simulink model "uz_codegen_mtpa_me"  (R2022b)
settings: Solver=FixedStepDiscrete  StartTime=0.0  StopTime=50  RelTol=1e-3  EnableMultiTasking=on
PreLoadFcn:
  | uz_setCodegenPaths
model workspace (MATLAB code in the model file):
  | cmdLim = Simulink.Parameter;
  | cmdLim.Value = 15;
  | cmdLim.Description = 'Limit for controlling the maximum surface command angle.';
  | cmdLim.Min = 0;
  | cmdLim.Max = 90;
  | cmdLim.DocUnits = 'deg';
  | 
  | dispGain = Simulink.Parameter;
  | dispGain.Value = 0.75;
  | dispGain.Description = 'Gain applied to the displacement error.';
  | dispGain.Min = 0;
  | dispGain.Max = [];
  | dispGain.DocUnits = 'deg/sec/deg';
  | 
  | dispLim = Simulink.Parameter;
  | dispLim.Value = 30;
  | dispLim.Description = 'Limit for controlling the maximum commanded angle.';
  | dispLim.Min = 0;
  | dispLim.Max = 180;
  | dispLim.DocUnits = 'deg';
  | 
  | intGain = Simulink.Parameter;
  | intGain.Value = 0.5;
  | intGain.Description = 'Gain applied to the integral error.';
  | intGain.Min = 0;
  | intGain.Max = [];
  | intGain.DocUnits = 'deg/sec/deg/sec';
  | 
  | intLim = Simulink.Parameter;
  | intLim.Value = 5;
  | intLim.Description = 'Limit for controlling the maximum commanded angle.';
  | intLim.Min = 0;
  | intLim.Max = 90;
  | intLim.DocUnits = 'deg';
  | 
  | rateGain = Simulink.Parameter;
  | rateGain.Value = 2;
  | rateGain.Description = 'Gain applied to the rate error.';
  | rateGain.Min = 0;
  | rateGain.Max = [];
  | rateGain.DocUnits = 'deg/deg/sec';
  | 
  | rateLim = Simulink.Parameter;
  | rateLim.Value = 6;
  | rateLim.Description = 'Limit for controlling the maximum commanded angle.';
  | rateLim.Min = 0;
  | rateLim.Max = 180;
  | rateLim.DocUnits = 'deg/sec';
  | 
  | hdgGain = Simulink.Parameter;
  | hdgGain.Value = 0.015;
undefined symbols (not defined in the file or in its folder): id_ME, id_MTPA, iq_ME, iq_MTPA, M_Mi_ME, M_Mi_MTPA, omega_ME
settings Model: RequirementInfo={} %GIDa_fe9045fd_0412_4b6e_8206_617cc20e6fde  FPTRunName=Active  Creator=ts  LastModifiedBy=Nina Diringer
settings SolverCC: AlgebraicLoopSolver=TrustRegion  PositivePriorityOrder=on  AutoInsertRateTranBlk=on
settings DataIOCC: SaveOutput=off  SignalLogging=off  DSMLogging=off  SaveTime=off
settings OptimizationCC: DefaultParameterBehavior=Inlined  UseDivisionForNetSlopeComputation=on  GainParamInheritBuiltInType=on  UseFloatMulNetSlope=on  UseSpecifiedMinMax=on  InlineInvariantSignals=on  PassReuseOutputArgsAs=Individual arguments  NoFixptDivByZeroProtection=on  EfficientFloat2IntCast=on  LifeSpan=1  MaxStackSize=64  OptimizeBlockOrder=speed  DifferentSizesBufferReuse=on  EfficientTunableParamExpr=on
settings DebuggingCC: UnconnectedInputMsg=warning  UnconnectedOutputMsg=warning  UnconnectedLineMsg=warning  AllowSymbolicDim=off  SFUnexpectedBacktrackingDiag=warning  SFNoUnconditionalDefaultTransitionDiag=warning  SFExecutionAtInitializationDiag=none  SFMachineParentedDataDiag=warning  ArithmeticOperatorsInVariantConditions=warning
settings HardwareCC: ProdBitPerPointer=32  ProdBitPerSizeT=32  ProdBitPerPtrDiffT=32  ProdLargestAtomicInteger=Long  ProdLargestAtomicFloat=Double  ProdWordSize=32  ProdLongLongMode=on  ProdHWDeviceType=ARM Compatible->ARM Cortex-R  HardwareBoardFeatureSet=SoCBlockset
settings ModelReferenceCC: EnableRefExpFcnMdlSchedulingChecks=on
settings SFSimCC: MATLABDynamicMemAlloc=off
settings RTWCC: Description=Embedded Coder  SystemTargetFile=ert.tlc  GenCodeOnly=on  TemplateMakefile=ert_default_tmf  GenerateReport=on  BuildConfiguration=Faster Runs  IncludeHyperlinkInReport=on  GenerateCodeMetricsReport=on  CheckMdlBeforeBuild=Warning  DLArmComputeVersion=19.05
settings CodeAppCC: ForceParamTrailComments=on  IgnoreCustomStorageClasses=off  OperatorAnnotations=on  SimulinkDataObjDesc=on  SFDataObjDesc=on  MATLABFcnDesc=on  CustomSymbolStrGlobalVar=rt$N$M  CustomSymbolStrType=$N$M  CustomSymbolStrFcn=$N$M$F  CustomSymbolStrMacro=$N$M  InsertBlockDesc=on  StateflowObjectComments=on  MATLABSourceComments=on  EnableCustomComments=on  ReqsInCode=on
settings ERTTargetCC: TargetLangStandard=C99 (ISO)  CodeReplacementLibrary=GNU C99 extensions  MultiwordLength=2048  IncludeMdlTerminateFcn=off  CombineSignalStateStructs=on  SuppressErrorStatus=on  IncludeFileDelimiter=UseQuote  SupportAbsoluteTime=off  CodeInterfacePackaging=Reusable function  SupportNonFinite=off  RemoveResetFunc=off  InlinedParameterPlacement=NonHierarchical  MultiInstanceErrorCode=Warning  RootIOFormat=Part of model data structure  ERTCustomFileTemplate=example_file_process.tlc  GlobalDataDefinition=InSourceFile  GlobalDataReference=InSourceFile  ERTFilePackagingFormat=CompactWithDataFile
settings ConfigComp: CovScope=ReferencedModels  CovSaveName=covdata_rollAP  CovMetricSettings=dcmtrwe  CovHTMLOptions=-sRT=1 -aTS=1 -bRG=1 -bTC=1 -hTR=1 -nFC=0 -scm=1 -bcm=1 -xEv=0  CovSaveCumulativeToWorkspaceVar=on  CovSaveSingleToWorkspaceVar=on  CovCumulativeVarName=covCumulativeData_rollAP  CovReportOnPause=off  CovExternalEMLEnable=off  CovSFcnEnable=off

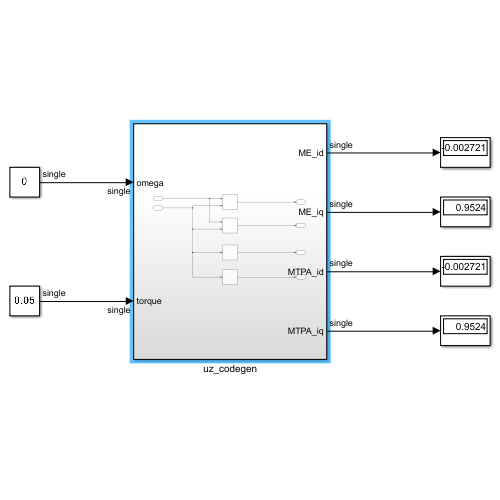
[thumbnail: Simulink's stored preview of the top-level diagram]
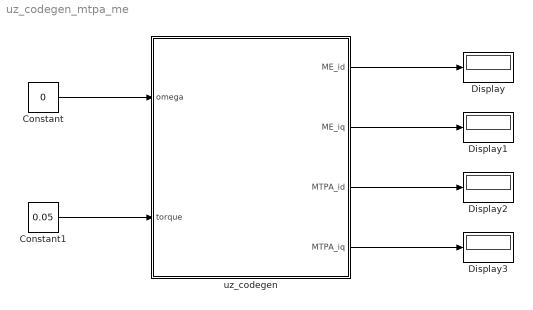
== system uz_codegen_mtpa_me ==
  Constant : Constant  Value=0  OutDataTypeStr=single  SampleTime=1/10000
  Constant1 : Constant  Value=0.05  OutDataTypeStr=single  SampleTime=1/10000
  Display{,1..3} (4 alike) : Display
  uz_codegen : Subsystem
  wires:
  Constant/1 -> uz_codegen/1(omega)
  Constant1/1 -> uz_codegen/2(torque)
  uz_codegen/1(ME_id) -> Display/1
  uz_codegen/2(ME_iq) -> Display1/1
  uz_codegen/4(MTPA_iq) -> Display3/1
  uz_codegen/3(MTPA_id) -> Display2/1

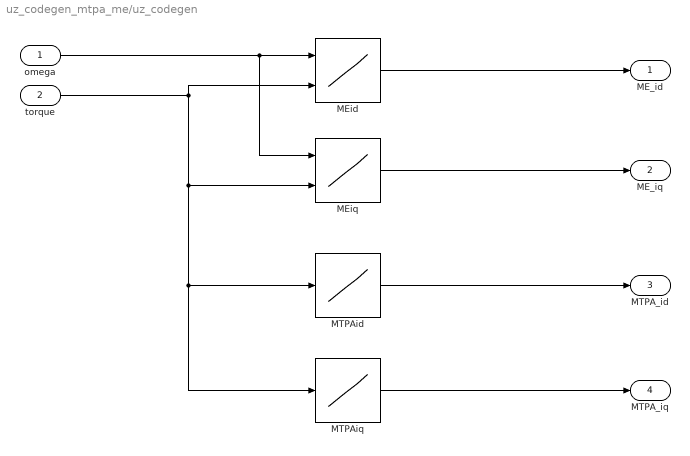
== system uz_codegen_mtpa_me/uz_codegen ==
  omega : Inport  OutDataTypeStr=single
  torque : Inport  Port=2  OutDataTypeStr=single
  MEid : Lookup_n-D  BreakpointsForDimension1=omega_ME  BreakpointsForDimension2=M_Mi_ME  Table=id_ME  InternalRulePriority=Speed  RndMeth=Simplest
      settings: InputPortMap=u0,u1
  MEiq : Lookup_n-D  BreakpointsForDimension1=omega_ME  BreakpointsForDimension2=M_Mi_ME  Table=iq_ME  InternalRulePriority=Speed  RndMeth=Simplest
      settings: InputPortMap=u0,u1
  MTPAid : Lookup_n-D  NumberOfTableDimensions=1  BreakpointsForDimension1=M_Mi_MTPA  Table=id_MTPA  InternalRulePriority=Speed  RndMeth=Simplest
  MTPAiq : Lookup_n-D  NumberOfTableDimensions=1  BreakpointsForDimension1=M_Mi_MTPA  Table=iq_MTPA  InternalRulePriority=Speed  RndMeth=Simplest
  ME_id : Outport  VectorParamsAs1DForOutWhenUnconnected=off
  ME_iq : Outport  Port=2  VectorParamsAs1DForOutWhenUnconnected=off
  MTPA_id : Outport  Port=3  VectorParamsAs1DForOutWhenUnconnected=off
  MTPA_iq : Outport  Port=4  VectorParamsAs1DForOutWhenUnconnected=off
  wires:
  omega/1 -> MEiq/1, MEid/1
  MEid/1 -> ME_id/1
  MEiq/1 -> ME_iq/1
  torque/1 -> MEiq/2, MTPAiq/1, MTPAid/1, MEid/2
  MTPAid/1 -> MTPA_id/1
  MTPAiq/1 -> MTPA_iq/1
